simulink model "Pid"  (R2018b)
settings: Solver=VariableStepAuto  StartTime=0.0  StopTime=10.0  RelTol=1e-3
undefined symbols (not defined in the file): parameter
settings Model: Creator=giga4  LastModifiedBy=giga4

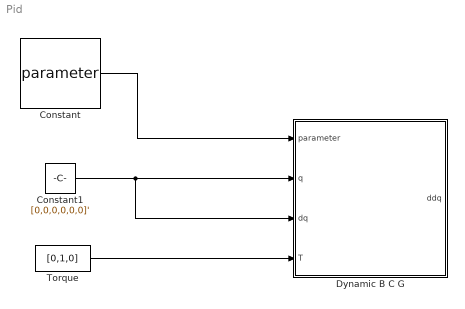
== system Pid ==
  Constant : Constant  Value=parameter
  Constant1 : Constant  Value=[0,0,0,0,0,0]'
  Dynamic B C G : MATLAB Function  TreatAsAtomicUnit=on
  Torque : Constant  Value=[0,1,0]
  wires:
  Constant/1 -> Dynamic B C G/1(parameter)
  Constant1/1 -> Dynamic B C G/3(dq), Dynamic B C G/2(q)
  Torque/1 -> Dynamic B C G/4(T)

== matlab function Pid/Dynamic B C G ==
  data: parameter input; q input; ddq output; dq input; T input
function ddq = Dynamic(parameter,q,dq,T)

[B,C,G] = generatore_dinamica(parameter,q,dq);

Q = [0,0,0,T(1),T(2),T(3)]';

ddq = B\(Q-C*dq-G);

end
